simulink library "CTRL_TRGT_YRDES"  (R2023b)
settings: Solver=VariableStepAuto  StartTime=0.0  StopTime=10.0  RelTol=1e-3
libraries: VUT_lib x1
settings Model: Creator=blatak  LastModifiedBy=blatak

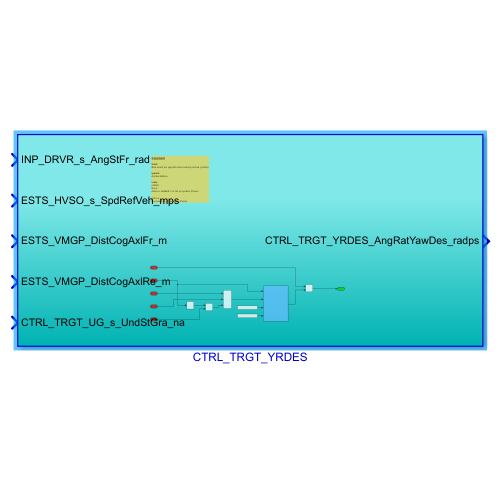
[thumbnail: Simulink's stored preview of the top-level diagram]
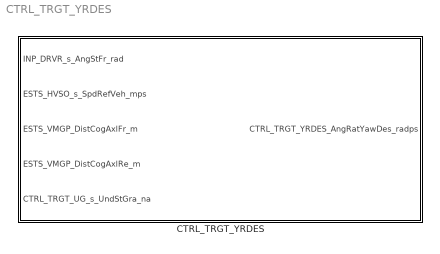
== system CTRL_TRGT_YRDES ==
  CTRL_TRGT_YRDES : Subsystem

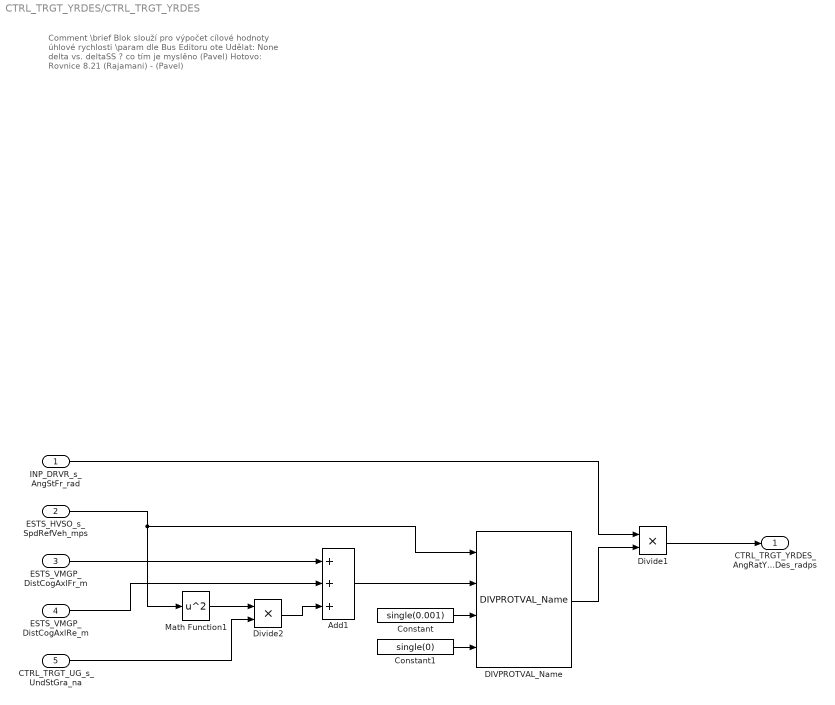
== system CTRL_TRGT_YRDES/CTRL_TRGT_YRDES ==
  note: Comment
      |
      | \brief
      | Blok slouží pro výpočet cílové hodnoty úhlové rychlosti
      |
      | \param
      | dle Bus Editoru
      |
      | \note
      | Udělat:
      | None
      | delta vs. deltaSS ? co tím je myslěno (Pavel)
      |
      | Hotovo:
      | Rovnice 8.21 (Rajamani) - (Pavel)
  INP_DRVR_s_AngStFr_rad : Inport
  ESTS_HVSO_s_SpdRefVeh_mps : Inport  Port=2
  ESTS_VMGP_DistCogAxlFr_m : Inport  Port=3
  ESTS_VMGP_DistCogAxlRe_m : Inport  Port=4
  CTRL_TRGT_UG_s_UndStGra_na : Inport  Port=5
  Add1 : Sum  Inputs=+++
  Constant : Constant  Value=single(0.001)
  Constant1 : Constant  Value=single(0)
  DIVPROTVAL_Name : VUT_lib/DIVPROTVAL_Name  SystemSampleTime=-1  VariantActivationTime=update diagram  AllowFlexibleInterface=on  Latency=0  AutoFrameSizeCalculation=off
  Divide1 : Product  Inputs=**
  Divide2 : Product  Inputs=**
  Math Function1 : Math  Operator=square
  CTRL_TRGT_YRDES_AngRatYawDes_radps : Outport
  wires:
  ESTS_VMGP_DistCogAxlRe_m/1 -> Add1/2
  Divide2/1 -> Add1/3
  Add1/1 -> DIVPROTVAL_Name/2
  CTRL_TRGT_UG_s_UndStGra_na/1 -> Divide2/2
  INP_DRVR_s_AngStFr_rad/1 -> Divide1/1
  ESTS_VMGP_DistCogAxlFr_m/1 -> Add1/1
  ESTS_HVSO_s_SpdRefVeh_mps/1 -> DIVPROTVAL_Name/1, Math Function1/1
  Math Function1/1 -> Divide2/1
  DIVPROTVAL_Name/1 -> Divide1/2
  Divide1/1 -> CTRL_TRGT_YRDES_AngRatYawDes_radps/1
  Constant/1 -> DIVPROTVAL_Name/3
  Constant1/1 -> DIVPROTVAL_Name/4
